simulink model "q1"  (R2022a)
settings: Solver=ode45  StartTime=0.0  StopTime=10.0  RelTol=1e-3
libraries: dspstat3 x1
settings Model: Creator=Guilherme  LastModifiedBy=Guilherme

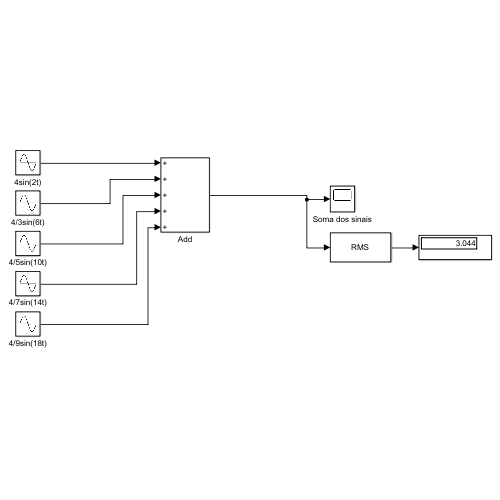
[thumbnail: Simulink's stored preview of the top-level diagram]
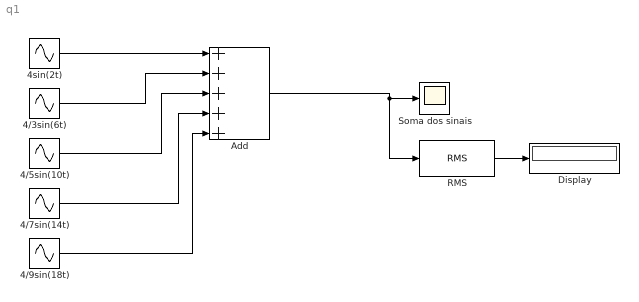
== system q1 ==
  4/3sin(6t) : Sin  Amplitude=4/3  Frequency=6  SampleTime=0
  4/5sin(10t) : Sin  Amplitude=4/5  Frequency=10  SampleTime=0
  4/7sin(14t) : Sin  Amplitude=4/7  Frequency=14  SampleTime=0
  4/9sin(18t) : Sin  Amplitude=4/9  Frequency=18  SampleTime=0
  4sin(2t) : Sin  Amplitude=4  Frequency=2  SampleTime=0
  Add : Sum  Inputs=+++++
  Display : Display
  RMS : dspstat3/RMS  run=off  directionMode=Each column  dimension=1  InputProcessing=Columns as channels (frame based)  reset_popup=None
  Soma dos sinais : Scope
  wires:
  4/9sin(18t)/1 -> Add/5
  4/7sin(14t)/1 -> Add/4
  4/5sin(10t)/1 -> Add/3
  4/3sin(6t)/1 -> Add/2
  4sin(2t)/1 -> Add/1
  Add/1 -> RMS/1, Soma dos sinais/1
  RMS/1 -> Display/1
